simulink model "Task_1_b"  (R2024b)
settings: Solver=ode4  StartTime=0.0  StopTime=50.0  FixedStep=0.01  RelTol=1e-3
settings Model: Creator=max  LastModifiedBy=max

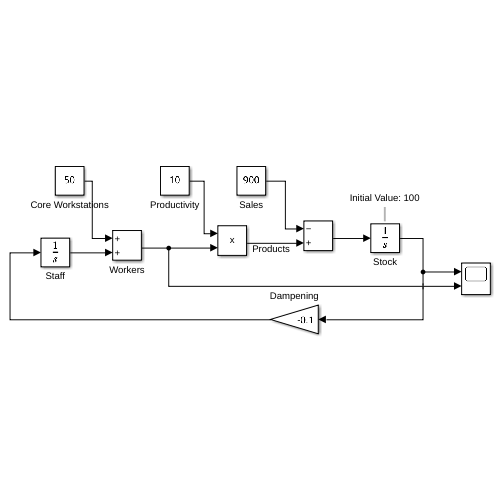
[thumbnail: Simulink's stored preview of the top-level diagram]
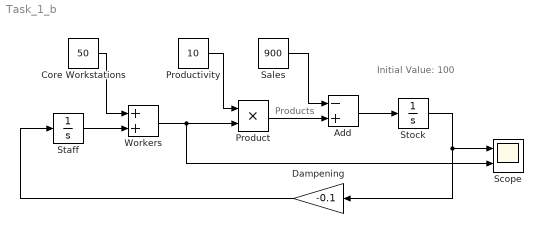
== system Task_1_b ==
  note: Products
  note: Initial Value: 100
  Add : Sum  Inputs=-+
  Core Workstations : Constant  Value=50
  Dampening : Gain  Gain=-0.1
  Product : Product
  Productivity : Constant  Value=10
  Sales : Constant  Value=900
  Scope : Scope  NumInputPorts=2
  Staff : Integrator
  Stock : Integrator  InitialCondition=100
  Workers : Sum
  wires:
  Add/1 -> Stock/1
  Sales/1 -> Add/1
  Product/1 -> Add/2
  Productivity/1 -> Product/1
  Stock/1 -> Dampening/1, Scope/1
  Dampening/1 -> Staff/1
  Staff/1 -> Workers/2
  Workers/1 -> Scope/2, Product/2
  Core Workstations/1 -> Workers/1
